simulink model "untitled3"  (R2018b)
settings: Solver=VariableStepAuto  StartTime=0.0  StopTime=5  RelTol=1e-3
libraries: commdigbbndpm3 x2, commsink2 x1, commutil2 x1, commfilt2 x1, commrandsrc3 x1
settings Model: Creator=nhat  LastModifiedBy=nhat

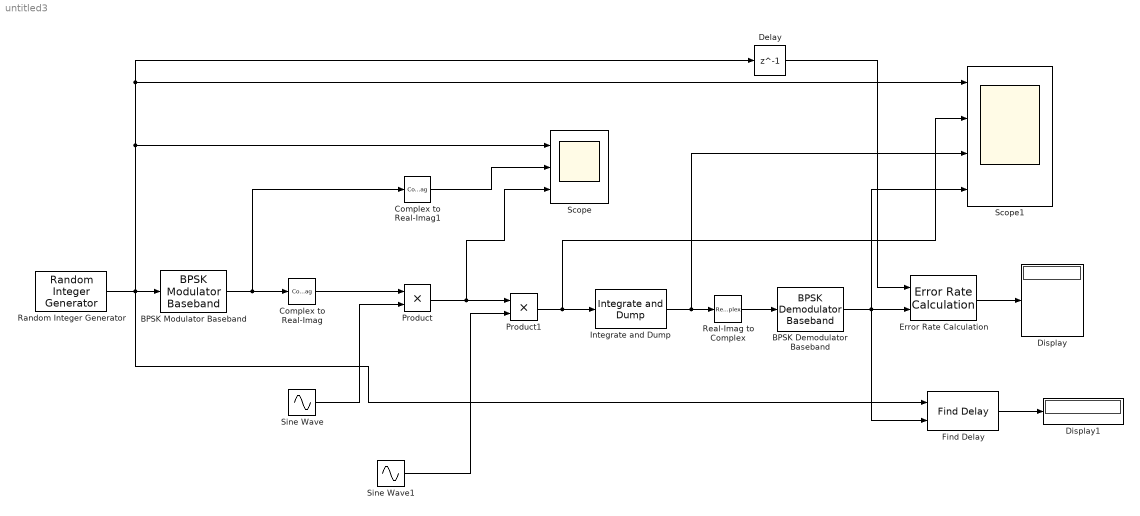
== system untitled3 ==
  BPSK Demodulator Baseband : commdigbbndpm3/BPSK Demodulator Baseband  DecType=Hard decision  VarSource=Dialog  Variance=1  Ph=0  outDtype=Inherit via internal rule  derotateFactorWordLen=16  derotateFactorDataTypeStr=Inherit: Same word length as input  derotateFactorLastDataTypeStr=Inherit: Same word length as input
  BPSK Modulator Baseband : commdigbbndpm3/BPSK Modulator Baseband  Ph=0  outDtype=double  outWordLen=16  outUDDataType=sfix(16)  outFracLenMode=Best precision  outFracLen=15  outDataTypeStr=double  outLastDataTypeStr=double
  Complex to Real-Imag : ComplexToRealImag  Output=Real
  Complex to Real-Imag1 : ComplexToRealImag  Output=Real
  Delay : Delay  DelayLength=1
  Display : Display
  Display1 : Display
  Error Rate Calculation : commsink2/Error Rate Calculation  N=0  st_delay=0  cp_mode=Entire frame  subframe=[]  PMode=Port  WsName=ErrorVec  RsMode2=off  stop=off  numErr=100  maxBits=1e6
  Find Delay : commutil2/Find Delay  corrLength=200  chgSigOP=off  stopUpdate=off  numConstDelay=3
      settings: SourceProductName=Communications System Toolbox  SourceProductBaseCode=CM
  Integrate and Dump : commfilt2/Integrate and Dump  obssamples=100  offsetsamples=0  nodump=off  roundingMode=Floor  overflowMode=off  outputDataTypeStr=Inherit: Same as accumulator  outputLastDataTypeStr=Inherit: Same as accumulator
      settings: SourceProductName=Communications System Toolbox
  Product : Product
  Product1 : Product
  Random Integer Generator : commrandsrc3/Random Integer Generator  SetSize=2  SeedSource=Auto  Seed=0  SampleTime=1/1000  SamplesPerFrame=1  OutputDataType=double  SimulateUsing=Interpreted execution
  Real-Imag to Complex : RealImagToComplex  Input=Real
  Scope : Scope  NumInputPorts=3
  Scope1 : Scope  NumInputPorts=4
  Sine Wave : Sin  Frequency=10000*2*pi  SampleTime=1/100000
  Sine Wave1 : Sin  Frequency=10000*pi*2  SampleTime=1/100000
  wires:
  Random Integer Generator/1 -> Scope/1, Scope1/1, Delay/1, Find Delay/1, BPSK Modulator Baseband/1
  BPSK Modulator Baseband/1 -> Complex to Real-Imag1/1, Complex to Real-Imag/1
  Complex to Real-Imag/1 -> Product/1
  Sine Wave/1 -> Product/2
  Product/1 -> Scope/3, Product1/1
  Sine Wave1/1 -> Product1/2
  Product1/1 -> Scope1/2, Integrate and Dump/1
  Integrate and Dump/1 -> Scope1/3, Real-Imag to Complex/1
  Real-Imag to Complex/1 -> BPSK Demodulator Baseband/1
  BPSK Demodulator Baseband/1 -> Scope1/4, Find Delay/2, Error Rate Calculation/2
  Error Rate Calculation/1 -> Display/1
  Delay/1 -> Error Rate Calculation/1
  Complex to Real-Imag1/1 -> Scope/2
  Find Delay/1 -> Display1/1
